simulink model "pcc_dynamic_model"  (R2021a)
settings: Solver=VariableStepAuto  StartTime=0.0  StopTime=10.0  MaxStep=0.005  RelTol=1e-3
libraries: simulink x3, simulink_extras x3
settings Model: Creator=maximilianstoelzle  LastModifiedBy=maximilianstoelzle

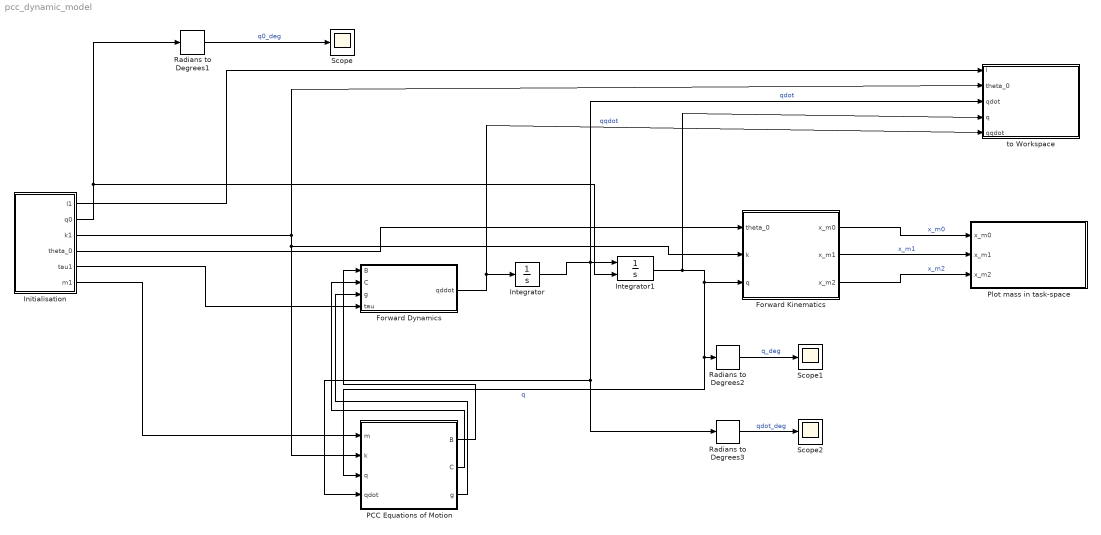
== system pcc_dynamic_model ==
  Forward Dynamics : MATLAB Function  TreatAsAtomicUnit=on
  Forward Kinematics : MATLAB Function  TreatAsAtomicUnit=on
  Initialisation : Subsystem
  Integrator : Integrator  InitialCondition=[0; 0; 0]
  Integrator1 : Integrator  InitialConditionSource=external
  PCC Equations of Motion : MATLAB Function  TreatAsAtomicUnit=on
  Plot mass in task-space : Subsystem
  Radians to Degrees1 : simulink_extras/Transformations/Radians to Degrees
  Radians to Degrees2 : simulink_extras/Transformations/Radians to Degrees
  Radians to Degrees3 : simulink_extras/Transformations/Radians to Degrees
  Scope : Scope
  Scope1 : Scope
  Scope2 : Scope
  to Workspace : Subsystem
  wires:
  Integrator/1 -> to Workspace/3(qdot), Radians to Degrees3/1, PCC Equations of Motion/4(qdot), Integrator1/1  "qdot"
  Integrator1/1 -> to Workspace/4(q), PCC Equations of Motion/3(q), Radians to Degrees2/1, Forward Kinematics/3(q)  "q"
  Radians to Degrees1/1 -> Scope/1  "q0_deg"
  Radians to Degrees2/1 -> Scope1/1  "q_deg"
  PCC Equations of Motion/1(B) -> Forward Dynamics/1(B)
  PCC Equations of Motion/2(C) -> Forward Dynamics/2(C)
  PCC Equations of Motion/3(g) -> Forward Dynamics/3(g)
  Forward Dynamics/1(qddot) -> to Workspace/5(qqdot), Integrator/1  "qqdot"
  Forward Kinematics/1(x_m0) -> Plot mass in task-space/1(x_m0)  "x_m0"
  Forward Kinematics/2(x_m1) -> Plot mass in task-space/2(x_m1)  "x_m1"
  Forward Kinematics/3(x_m2) -> Plot mass in task-space/3(x_m2)  "x_m2"
  Initialisation/3(k1) -> PCC Equations of Motion/2(k), Forward Kinematics/2(k), to Workspace/2(theta_0)
  Initialisation/2(q0) -> Radians to Degrees1/1, Integrator1/2
  Initialisation/1(l1) -> to Workspace/1(l)
  Initialisation/4(theta_0) -> Forward Kinematics/1(theta_0)
  Initialisation/5(tau1) -> Forward Dynamics/4(tau)
  Initialisation/6(m1) -> PCC Equations of Motion/1(m)
  Radians to Degrees3/1 -> Scope2/1  "qdot_deg"

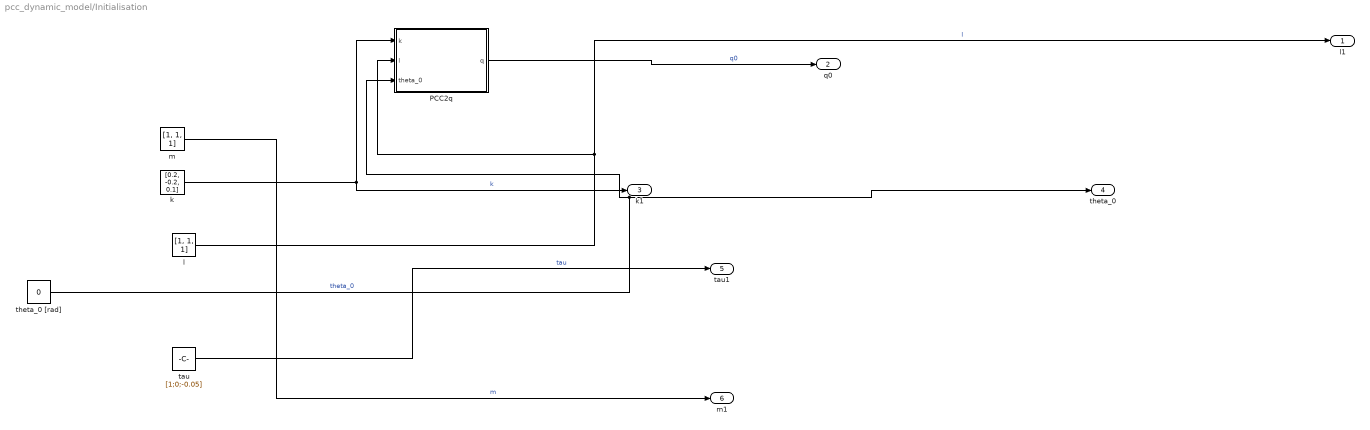
== system pcc_dynamic_model/Initialisation ==
  PCC2q : MATLAB Function  TreatAsAtomicUnit=on
  k : Constant  Value=[0.2, -0.2, 0.1]
  l : Constant  Value=[1, 1, 1]
  m : Constant  Value=[1, 1, 1]
  tau : Constant  Value=[1;0;-0.05]
  theta_0 [rad] : Constant  Value=0
  l1 : Outport
  q0 : Outport  Port=2
  k1 : Outport  Port=3
  theta_0 : Outport  Port=4
  tau1 : Outport  Port=5
  m1 : Outport  Port=6
  wires:
  tau/1 -> tau1/1  "tau"
  PCC2q/1(q) -> q0/1  "q0"
  k/1 -> k1/1, PCC2q/1(k)  "k"
  m/1 -> m1/1  "m"
  theta_0 [rad]/1 -> theta_0/1, PCC2q/3(theta_0)  "theta_0"
  l/1 -> l1/1, PCC2q/2(l)  "l"

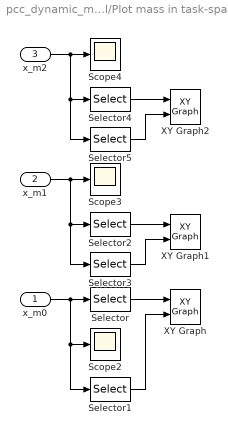
== system pcc_dynamic_model/Plot mass in task-space ==
  x_m0 : Inport
  x_m1 : Inport  Port=2
  x_m2 : Inport  Port=3
  Scope2 : Scope
  Scope3 : Scope
  Scope4 : Scope
  Selector : Selector  InputPortWidth=2  IndexOptions=Index vector (dialog)  Indices=[1]  OutputSizes=1
  Selector1 : Selector  InputPortWidth=2  IndexOptions=Index vector (dialog)  Indices=[2]  OutputSizes=1
  Selector2 : Selector  InputPortWidth=2  IndexOptions=Index vector (dialog)  Indices=[1]  OutputSizes=1
  Selector3 : Selector  InputPortWidth=2  IndexOptions=Index vector (dialog)  Indices=[2]  OutputSizes=1
  Selector4 : Selector  InputPortWidth=2  IndexOptions=Index vector (dialog)  Indices=[1]  OutputSizes=1
  Selector5 : Selector  InputPortWidth=2  IndexOptions=Index vector (dialog)  Indices=[2]  OutputSizes=1
  XY Graph : simulink/Sinks/XY Graph  xmin=-10  xmax=10  ymin=-10  ymax=10  st=-1
  XY Graph1 : simulink/Sinks/XY Graph  xmin=-10  xmax=10  ymin=-10  ymax=10  st=-1
  XY Graph2 : simulink/Sinks/XY Graph  xmin=-10  xmax=10  ymin=-10  ymax=10  st=-1
  wires:
  x_m2/1 -> Selector5/1, Selector4/1, Scope4/1
  Selector/1 -> XY Graph/1
  x_m1/1 -> Selector3/1, Selector2/1, Scope3/1
  Selector5/1 -> XY Graph2/2
  Selector3/1 -> XY Graph1/2
  Selector1/1 -> XY Graph/2
  x_m0/1 -> Scope2/1, Selector1/1, Selector/1
  Selector4/1 -> XY Graph2/1
  Selector2/1 -> XY Graph1/1

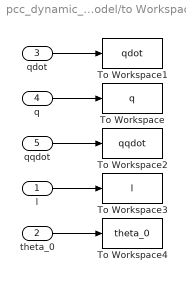
== system pcc_dynamic_model/to Workspace ==
  l : Inport
  theta_0 : Inport  Port=2
  qdot : Inport  Port=3
  q : Inport  Port=4
  qqdot : Inport  Port=5
  To Workspace : ToWorkspace  VariableName=q  SaveFormat=Timeseries  SampleTime=-1
  To Workspace1 : ToWorkspace  VariableName=qdot  SaveFormat=Timeseries  SampleTime=-1
  To Workspace2 : ToWorkspace  VariableName=qqdot  SaveFormat=Timeseries  SampleTime=-1
  To Workspace3 : ToWorkspace  VariableName=l  SaveFormat=Timeseries  SampleTime=-1
  To Workspace4 : ToWorkspace  VariableName=theta_0  SaveFormat=Timeseries  SampleTime=-1
  wires:
  theta_0/1 -> To Workspace4/1
  qdot/1 -> To Workspace1/1
  l/1 -> To Workspace3/1
  qqdot/1 -> To Workspace2/1
  q/1 -> To Workspace/1

== matlab function pcc_dynamic_model/Forward Kinematics ==
  data: theta_0 input; x_m0 output; k input; q input; x_m1 output; x_m2 output
function [x_m0, x_m1, x_m2] = forward_kinematics(theta_0, k, q)
    x_m0 = [(sin(q(1)) - sin(theta_0))/k(1); 
            -(cos(q(1)) - cos(theta_0))/k(1)];
    x_m1 = x_m0 + [(sin(q(2)) - sin(q(1)))/k(2); 
                   -(cos(q(2)) - cos(q(1)))/k(2)];
    x_m2 = x_m1 + [(sin(q(3)) - sin(q(2)))/k(3); 
                   -(cos(q(3)) - cos(q(2)))/k(3)];

end

== matlab function pcc_dynamic_model/Forward Dynamics ==
  data: B input; qddot output; C input; g input; tau input
function qddot  = forward_dynamics(B, C, g, tau)
    pinv_tol = 0.0001;
    qddot = pinv(B, pinv_tol)*(-C-g+tau);
end

== matlab function pcc_dynamic_model/Initialisation/PCC2q ==
  data: k input; q output; l input; theta_0 input
function q = pcc2q(k, l, theta_0)
    q = [theta_0 + k(1) * l(1);
         theta_0 + k(1) * l(1) + k(2) * l(2);
         theta_0 + k(1) * l(1) + k(2) * l(2) + k(3) * l(3)];
end

== matlab function pcc_dynamic_model/PCC Equations of Motion ==
  data: m input; B output; k input; q input; qdot input; C output; g output
function [B, C, g]  = pcc_eom(m, k, q, qdot)
    J_m0_P = [cos(q(1))/k(1), 0, 0;
              sin(q(1))/k(1), 0, 0];
    J_m1_P = [cos(q(1))*(1/k(1)-1/k(2)), cos(q(2))/k(2), 0;
              sin(q(1))*(1/k(1)-1/k(2)), sin(q(2))/k(2), 0];
    J_m2_P = [cos(q(1))*(1/k(1)-1/k(2)), cos(q(2))*(1/k(2)-1/k(3)), cos(q(3))/k(3);
              sin(q(1))*(1/k(1)-1/k(2)), sin(q(2))*(1/k(2)-1/k(3)), sin(q(3))/k(3)];
    Jdot_m0_P = [-sin(q(1))/k(1)*qdot(1), 0, 0;
                 cos(q(1))/k(1)*qdot(1), 0, 0];
    Jdot_m1_P = [-sin(q(1))*(1/k(1)-1/k(2))*qdot(1), cos(q(2))/k(2)*qdot(2), 0;
                 cos(q(1))*(1/k(1)-1/k(2)), sin(q(2))/k(2)*qdot(2), 0];
    Jdot_m2_P = [-sin(q(1))*(1/k(1)-1/k(2))*qdot(1), -sin(q(2))*(1/k(2)-1/k(3))*qdot(2), cos(q(3))/k(3)*qdot(3);
                 cos(q(1))*(1/k(1)-1/k(2))*qdot(1), cos(q(2))*(1/k(2)-1/k(3))*qdot(2), sin(q(3))/k(3)*qdot(3)];
    B = J_m0_P'*m(1)*J_m0_P + J_m1_P'*m(2)*J_m1_P + J_m2_P'*m(3)*J_m2_P;
    C = (Jdot_m0_P'*m(1)*J_m0_P + Jdot_m1_P'*m(2)*J_m1_P + Jdot_m2_P'*m(3)*J_m2_P)*qdot;
    g = [0; 0; 0];
end
